simulink model "Stabilisation_trajectoire_constante"  (R2022b)
settings: Solver=ode45  StartTime=0.0  StopTime=80  RelTol=1e-3  EnableMultiTasking=on
settings Model: Creator=Dalil  LastModifiedBy=33605
settings SolverCC: AlgebraicLoopSolver=TrustRegion
settings DataIOCC: LimitDataPoints=on  SaveFormat=Array  ReturnWorkspaceOutputs=off
settings OptimizationCC: ExpressionDepthLimit=2147483647  LifeSpan=inf
settings DebuggingCC: UnderspecifiedInitializationDetection=Classic  MergeDetectMultiDrivingBlocksExec=none  SolverPrmCheckMsg=warning  UnconnectedInputMsg=warning  UnconnectedOutputMsg=warning  UnconnectedLineMsg=warning  StateNameClashWarn=warning  SFUnexpectedBacktrackingDiag=warning  SFNoUnconditionalDefaultTransitionDiag=warning  SFExecutionAtInitializationDiag=none  SFMachineParentedDataDiag=warning  ArithmeticOperatorsInVariantConditions=warning
settings HardwareCC: ProdBitPerPointer=32  ProdBitPerSizeT=32  ProdBitPerPtrDiffT=32  ProdLargestAtomicFloat=None  ProdIntDivRoundTo=Undefined  ProdEndianess=Unspecified  ProdWordSize=32  ProdHWDeviceType=32-bit Generic
settings ModelReferenceCC: EnableRefExpFcnMdlSchedulingChecks=on  PropagateSignalLabelsOutOfModel=off
settings SFSimCC: SimUseLocalCustomCode=off  CustomCodeUndefinedFunction=UseInterfaceOnly
settings RTWCC: RTWUseLocalCustomCode=off
settings CodeAppCC: StateflowObjectComments=on
settings GRTTargetCC: TargetLangStandard=C89/C90 (ANSI)
settings ConfigComp: CovMetricSettings=dw  CovSaveCumulativeToWorkspaceVar=on  CovSaveSingleToWorkspaceVar=on  CovExternalEMLEnable=off

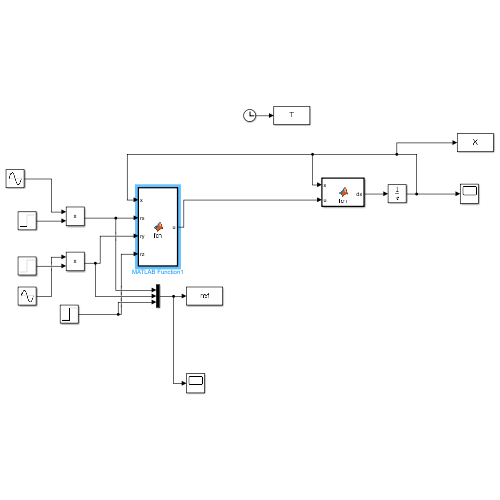
[thumbnail: Simulink's stored preview of the top-level diagram]
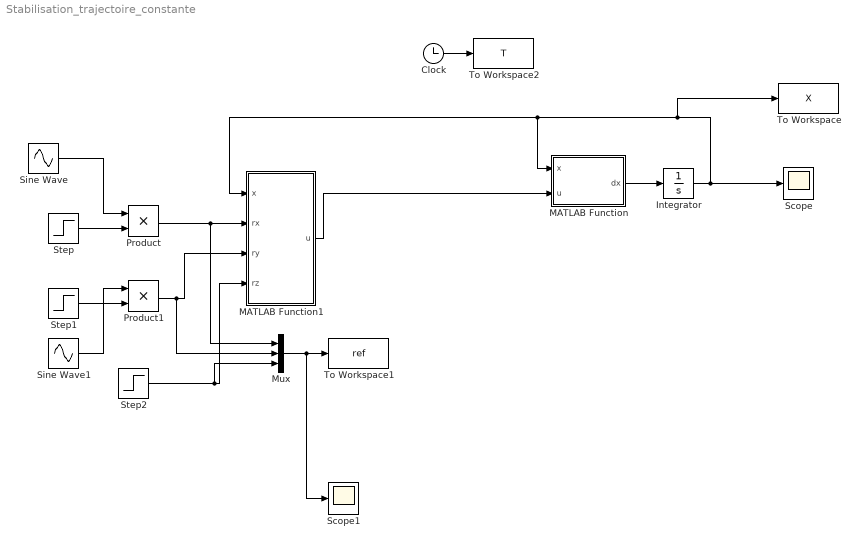
== system Stabilisation_trajectoire_constante ==
  Clock : Clock
  Integrator : Integrator  InitialCondition=0.1*[1 1 1 1 1 1 1 1 1 1 1 1]
  MATLAB Function : MATLAB Function  TreatAsAtomicUnit=on
  MATLAB Function1 : MATLAB Function  TreatAsAtomicUnit=on
  Mux : Mux  Inputs=3
  Product : Product
  Product1 : Product
  Scope : Scope
  Scope1 : Scope
  Sine Wave : Sin  Frequency=0.1  SampleTime=0
  Sine Wave1 : Sin  Frequency=0.1  Phase=pi/2  SampleTime=0
  Step : Step  Time=10  SampleTime=0
  Step1 : Step  Time=20  SampleTime=0
  Step2 : Step  Time=0  SampleTime=0
  To Workspace : ToWorkspace  VariableName=X  SampleTime=-1
  To Workspace1 : ToWorkspace  VariableName=ref  SampleTime=-1
  To Workspace2 : ToWorkspace  VariableName=T  SampleTime=-1
  wires:
  MATLAB Function/1(dx) -> Integrator/1
  Integrator/1 -> To Workspace/1, MATLAB Function/1(x), MATLAB Function1/1(x), Scope/1
  MATLAB Function1/1(u) -> MATLAB Function/2(u)
  Step2/1 -> Mux/3, MATLAB Function1/4(rz)
  Mux/1 -> Scope1/1, To Workspace1/1
  Clock/1 -> To Workspace2/1
  Step/1 -> Product/2
  Sine Wave/1 -> Product/1
  Product/1 -> Mux/1, MATLAB Function1/2(rx)
  Step1/1 -> Product1/2
  Product1/1 -> Mux/2, MATLAB Function1/3(ry)
  Sine Wave1/1 -> Product1/1

== matlab function Stabilisation_trajectoire_constante/MATLAB Function1 ==
  data: x input; u output; rx input; ry input; rz input
function u = fcn(x,rx,ry,rz)
%#codegen


u = zeros(6,1);

g  = 9.81;

% les moments inirtiels 
Ixx=7.5*10^-3;
Iyy=7.5*10^-3;
Izz=1.3*10^-3;

k1 = 2; k2 = 3;
k3 = 3; k4 = 5;
k5 = 2; k6 = 4;
k7 = 2; k8 = 3;
k9 = 2; k10 = 6;
k11 = 2; k12 = 3;

% les coeficients 
a1=((Iyy-Izz)/Ixx);
a2=((Izz-Ixx)/Iyy);
a3=((Ixx-Iyy)/Izz);


u(1) = -(x(12)*x(4)-x(10)*x(6)-g*sin(x(9)))-k1*(x(1)-rx)-k2*x(2);
u(2) = -(x(8)*x(6)-x(12)*x(2)+g*sin(x(7))*cos(x(9)))-k3*(x(3)-ry)-k4*x(4);
u(3) = -(x(10)*x(2)-x(8)*x(4)+g*cos(x(7))*cos(x(9)))-k5*(x(5)-rz)-k6*x(6);
u(4) = -(a1*x(12)*x(10))-k7*x(7)-k8*x(8);
u(5) = -a2*x(12)*x(8)-k9*x(9)-k10*x(10);
u(6) = -a3*x(8)*x(10)-k11*x(11)-k12*x(12);

== matlab function Stabilisation_trajectoire_constante/MATLAB Function ==
  data: x input; u input; dx output
function dx = fcn(x,u)
%#codegen

g  = 9.81;

% les moments inirtiels 
Ixx=7.5*10^-3;
Iyy=7.5*10^-3;
Izz=1.3*10^-3;


% les coeficients 
a1=((Iyy-Izz)/Ixx);
a2=((Izz-Ixx)/Iyy);
a3=((Ixx-Iyy)/Izz);

dx = zeros(12,1);

dx(1) = x(2);
dx(2) = x(12)*x(4)-x(10)*x(6)-g*sin(x(9))+u(1);
dx(3) = x(4);
dx(4) = x(8)*x(6)-x(12)*x(2)+g*sin(x(7))*cos(x(9))+u(2);
dx(5) = x(6);
dx(6) = x(10)*x(2)-x(8)*x(4)+g*cos(x(7))*cos(x(9))+u(3);
dx(7) = x(8);
dx(8) = a1*x(12)*x(10)+u(4);
dx(9) = x(10);
dx(10) = a2*x(12)*x(8)+u(5);
dx(11) = x(12);
dx(12) = a3*x(8)*x(10)+u(6);
